simulink model "Pendulum"  (R2024b)
settings: Solver=FixedStepAuto  StartTime=0.0  StopTime=10  FixedStep=0.001  RelTol=1e-3
values from neighbouring files (symbols this model uses):
  b_1 = 0.1    [main.m]
  b_2 = 0.1    [main.m]
  Ia_z1 = 0.05    [main.m]
  Ip_x2 = 0.02    [main.m]
  Ip_y2 = 0.015    [main.m]
  l = 1.0    (= 1)    [main.m]
  m_p = 0.5    [main.m]
  phi_dot_dot_sat = 100    [main.m]
  phi_dot_dot_threshold = 1e-10    [main.m]
  r = 0.3    [main.m]
  tau_a_sat = inf    [main.m]
  tau_a_threshold = 1e-10    [main.m]
  theta_dot_dot_sat = 100    [main.m]
  theta_dot_dot_threshold = 1e-10    [main.m]
settings Model: Creator=sipak  LastModifiedBy=sipak

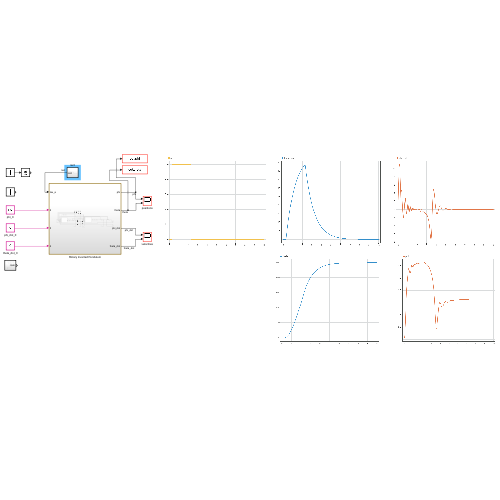
[thumbnail: Simulink's stored preview of the top-level diagram]
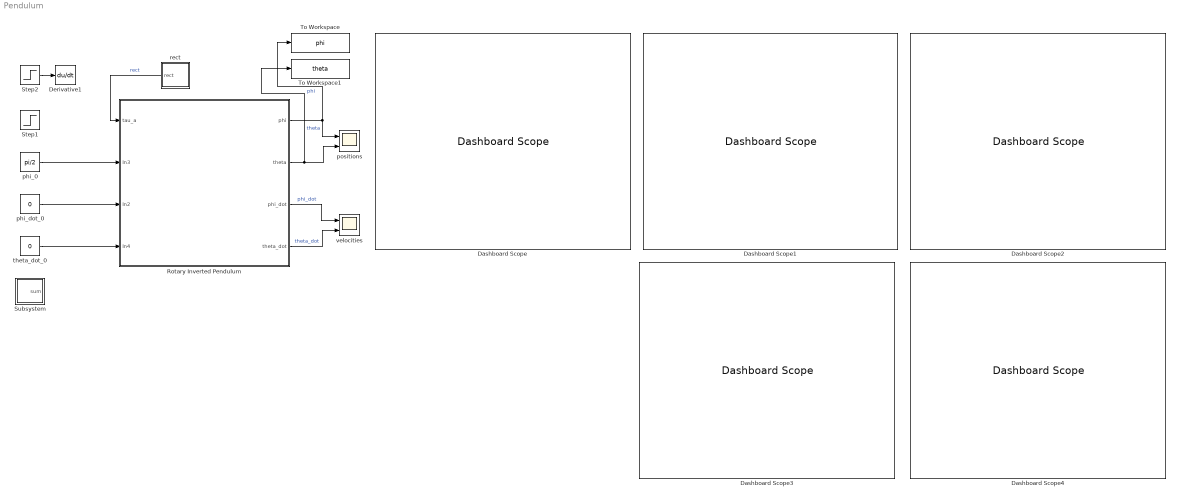
== system Pendulum ==
  Dashboard Scope{,1..4} (5 alike) : DashboardScope
  Derivative1 : Derivative
  Rotary Inverted Pendulum : Subsystem
  Step1 : Step  After=5  SampleTime=0
  Step2 : Step  After=1e10  SampleTime=0
  Subsystem : Subsystem
  To Workspace : ToWorkspace  VariableName=phi  SampleTime=-1
      settings: Save2DSignal=2-D array (concatenate along first dimension)
  To Workspace1 : ToWorkspace  VariableName=theta  SampleTime=-1
      settings: Save2DSignal=2-D array (concatenate along first dimension)
  phi_0 : Constant  Value=pi/2
  phi_dot_0 : Constant  Value=0
  positions : Scope  NumInputPorts=2
  rect : Subsystem
  theta_dot_0 : Constant  Value=0
  velocities : Scope  NumInputPorts=2
  wires:
  phi_dot_0/1 -> Rotary Inverted Pendulum/3(In2)
  Rotary Inverted Pendulum/2(theta) -> To Workspace1/1, positions/2  "theta"
  Rotary Inverted Pendulum/1(phi) -> To Workspace/1, positions/1  "phi"
  phi_0/1 -> Rotary Inverted Pendulum/2(In3)
  Rotary Inverted Pendulum/3(phi_dot) -> velocities/1  "phi_dot"
  Rotary Inverted Pendulum/4(theta_dot) -> velocities/2  "theta_dot"
  theta_dot_0/1 -> Rotary Inverted Pendulum/4(In4)
  Step2/1 -> Derivative1/1
  rect/1(rect) -> Rotary Inverted Pendulum/1(tau_a)  "rect"

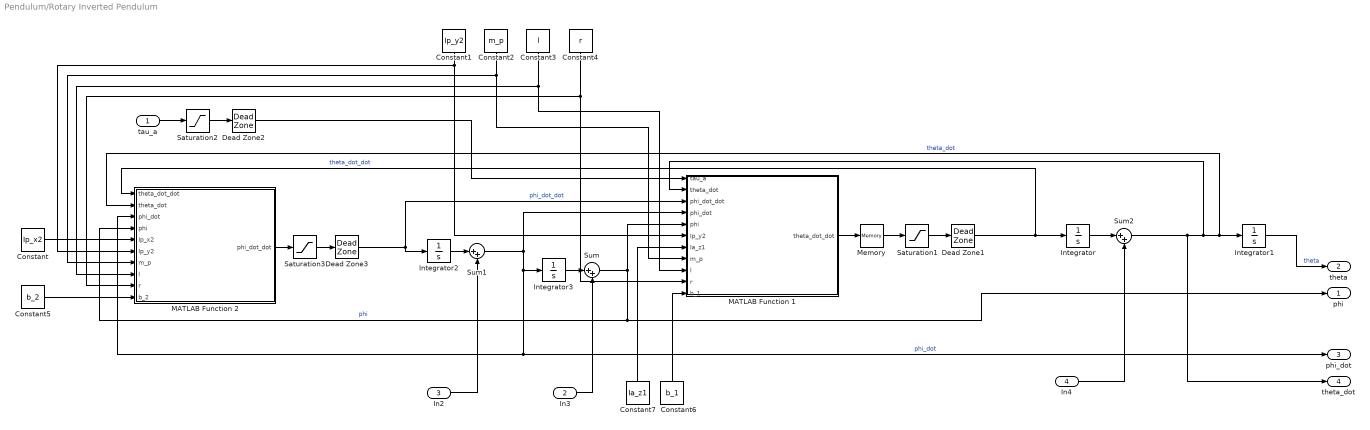
== system Pendulum/Rotary Inverted Pendulum ==
  tau_a : Inport
  In3 : Inport  Port=2
  In2 : Inport  Port=3
  In4 : Inport  Port=4
  Constant : Constant  Value=Ip_x2
  Constant1 : Constant  Value=Ip_y2
  Constant2 : Constant  Value=m_p
  Constant3 : Constant  Value=l
  Constant4 : Constant  Value=r
  Constant5 : Constant  Value=b_2
  Constant6 : Constant  Value=b_1
  Constant7 : Constant  Value=Ia_z1
  Dead Zone1 : DeadZone  LowerValue=-theta_dot_dot_threshold  UpperValue=theta_dot_dot_threshold
  Dead Zone2 : DeadZone  LowerValue=-tau_a_threshold  UpperValue=tau_a_threshold
  Dead Zone3 : DeadZone  LowerValue=-phi_dot_dot_threshold  UpperValue=phi_dot_dot_threshold
  Integrator{,1..3} (4 alike) : Integrator
  MATLAB Function 1 : MATLAB Function  TreatAsAtomicUnit=on
  MATLAB Function 2 : MATLAB Function  TreatAsAtomicUnit=on
  Memory : Memory
  Saturation1 : Saturate  UpperLimit=theta_dot_dot_sat  LowerLimit=-theta_dot_dot_sat
  Saturation2 : Saturate  UpperLimit=tau_a_sat  LowerLimit=-tau_a_sat
  Saturation3 : Saturate  UpperLimit=phi_dot_dot_sat  LowerLimit=-phi_dot_dot_sat
  Sum : Sum  Inputs=|++
  Sum1 : Sum  Inputs=|++
  Sum2 : Sum  Inputs=|++
  phi : Outport
  theta : Outport  Port=2
  phi_dot : Outport  Port=3
  theta_dot : Outport  Port=4
  wires:
  Integrator2/1 -> Sum1/1
  Integrator/1 -> Sum2/1
  Sum/1 -> phi/1, MATLAB Function 2/4(phi), MATLAB Function 1/5(phi)  "phi"
  MATLAB Function 2/1(phi_dot_dot) -> Saturation3/1
  In3/1 -> Sum/2
  tau_a/1 -> Saturation2/1
  Integrator3/1 -> Sum/1
  In4/1 -> Sum2/2
  In2/1 -> Sum1/2
  MATLAB Function 1/1(theta_dot_dot) -> Memory/1
  Integrator1/1 -> theta/1  "theta"
  Memory/1 -> Saturation1/1
  Sum1/1 -> phi_dot/1, MATLAB Function 2/3(phi_dot), Integrator3/1, MATLAB Function 1/4(phi_dot)  "phi_dot"
  Sum2/1 -> MATLAB Function 1/2(theta_dot), MATLAB Function 2/2(theta_dot), Integrator1/1, theta_dot/1  "theta_dot"
  Saturation2/1 -> Dead Zone2/1
  Dead Zone2/1 -> MATLAB Function 1/1(tau_a)
  Dead Zone3/1 -> MATLAB Function 1/3(phi_dot_dot), Integrator2/1  "phi_dot_dot"
  Saturation3/1 -> Dead Zone3/1
  Saturation1/1 -> Dead Zone1/1
  Dead Zone1/1 -> MATLAB Function 2/1(theta_dot_dot), Integrator/1  "theta_dot_dot"
  Constant/1 -> MATLAB Function 2/5(Ip_x2)
  Constant1/1 -> MATLAB Function 1/6(Ip_y2), MATLAB Function 2/6(Ip_y2)
  Constant2/1 -> MATLAB Function 1/8(m_p), MATLAB Function 2/7(m_p)
  Constant3/1 -> MATLAB Function 2/8(l), MATLAB Function 1/9(l)
  Constant4/1 -> MATLAB Function 1/10(r), MATLAB Function 2/9(r)
  Constant5/1 -> MATLAB Function 2/10(b_2)
  Constant7/1 -> MATLAB Function 1/7(Ia_z1)
  Constant6/1 -> MATLAB Function 1/11(b_1)

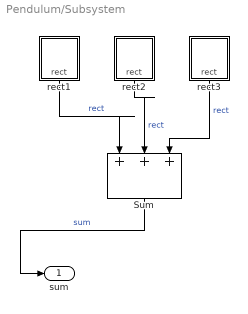
== system Pendulum/Subsystem ==
  Sum : Sum  Inputs=|+++
  rect1 : Subsystem
  rect2 : Subsystem
  rect3 : Subsystem
  sum : Outport
  wires:
  Sum/1 -> sum/1  "sum"
  rect1/1(rect) -> Sum/1  "rect"
  rect2/1(rect) -> Sum/2  "rect"
  rect3/1(rect) -> Sum/3  "rect"

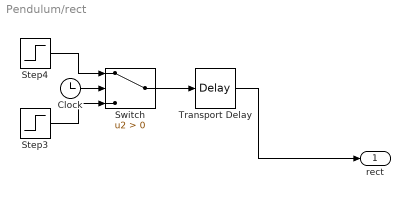
== system Pendulum/rect ==
  Clock : Clock
  Step3 : Step  After=5  SampleTime=0
  Step4 : Step  Time=2  Before=5  After=0  SampleTime=0
  Switch : Switch  Criteria=u2 > Threshold  SaturateOnIntegerOverflow=off  InputSameDT=off
  Transport Delay : TransportDelay  DelayTime=0.3
  rect : Outport
  wires:
  Clock/1 -> Switch/2
  Step3/1 -> Switch/3
  Switch/1 -> Transport Delay/1
  Step4/1 -> Switch/1
  Transport Delay/1 -> rect/1

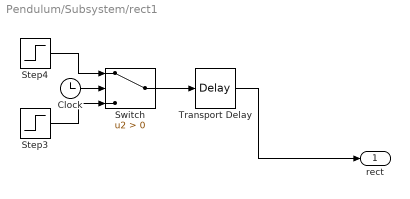
== system Pendulum/Subsystem/rect1 ==
  Clock : Clock
  Step3 : Step  After=5  SampleTime=0
  Step4 : Step  Time=2  Before=5  After=0  SampleTime=0
  Switch : Switch  Criteria=u2 > Threshold  SaturateOnIntegerOverflow=off  InputSameDT=off
  Transport Delay : TransportDelay
  rect : Outport
  wires:
  Transport Delay/1 -> rect/1
  Step4/1 -> Switch/1
  Switch/1 -> Transport Delay/1
  Step3/1 -> Switch/3
  Clock/1 -> Switch/2

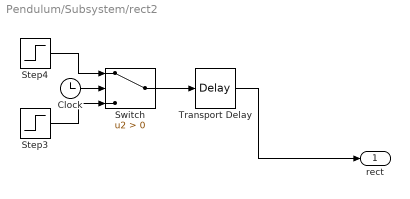
== system Pendulum/Subsystem/rect2 ==
  Clock : Clock
  Step3 : Step  After=-5  SampleTime=0
  Step4 : Step  Time=2  Before=-5  After=0  SampleTime=0
  Switch : Switch  Criteria=u2 > Threshold  SaturateOnIntegerOverflow=off  InputSameDT=off
  Transport Delay : TransportDelay  DelayTime=4
  rect : Outport
  wires:
  Clock/1 -> Switch/2
  Step3/1 -> Switch/3
  Switch/1 -> Transport Delay/1
  Step4/1 -> Switch/1
  Transport Delay/1 -> rect/1

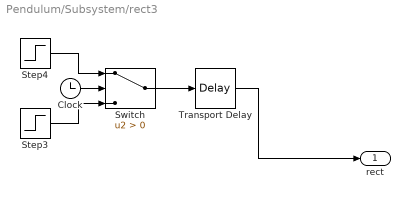
== system Pendulum/Subsystem/rect3 ==
  Clock : Clock
  Step3 : Step  After=5  SampleTime=0
  Step4 : Step  Time=2  Before=5  After=0  SampleTime=0
  Switch : Switch  Criteria=u2 > Threshold  SaturateOnIntegerOverflow=off  InputSameDT=off
  Transport Delay : TransportDelay  DelayTime=7
  rect : Outport
  wires:
  Transport Delay/1 -> rect/1
  Step4/1 -> Switch/1
  Switch/1 -> Transport Delay/1
  Step3/1 -> Switch/3
  Clock/1 -> Switch/2

== matlab function Pendulum/Rotary Inverted Pendulum/MATLAB Function 2 ==
  data: theta_dot_dot input; phi_dot_dot output; theta_dot input; phi_dot input; phi input; Ip_x2 input; Ip_y2 input; m_p input; l input; r input; b_2 input
function phi_dot_dot = equation2(theta_dot_dot, theta_dot, phi_dot, phi, Ip_x2, Ip_y2, m_p, l, r, b_2)
    g = 9.81;  % Gravitational acceleration (m/s²)
    tau_p = 0;
    
    phi_dot_dot = (tau_p - ((1/2) * m_p * l * r * theta_dot_dot * cos(phi)) ...
                   + ((1/2) * theta_dot^2 * Ip_y2 * sin(2 * phi)) ...
                   + (m_p * g * (l / 2) * sin(phi)) ...
                   - (b_2 * phi_dot)) / Ip_x2;

== matlab function Pendulum/Rotary Inverted Pendulum/MATLAB Function 1 ==
  data: tau_a input; theta_dot_dot output; theta_dot input; phi_dot_dot input; phi_dot input; phi input; Ip_y2 input; Ia_z1 input; m_p input; l input; r input; b_1 input
function theta_dot_dot = equation1(tau_a, theta_dot, phi_dot_dot, phi_dot, phi, Ip_y2, Ia_z1, m_p, l, r, b_1)
    g = 9.81;  % Gravitational acceleration (m/s²)
    
    phi_dot_dot = 0; phi_dot = 0; phi = 0; % We assume that the pendulum dynamic has no effect on the motor 
    theta_dot_dot = (tau_a - (theta_dot * phi_dot * sin(2 * phi) * Ip_y2) ...
                     - ((1/2) * m_p * l * r * (phi_dot_dot * cos(phi) - phi_dot^2 * sin(phi))) ...
                     - (b_1 * theta_dot)) ...
                    / (Ia_z1 + Ip_y2 * sin(phi)^2 + m_p * r^2);
